simulink model "figura10"  (Simulink 8.8)
settings: Solver=ode45  StartTime=0.0  RelTol=1e-3  EnableMultiTasking=on
libraries: dsparch4 x1, dspsrcs4 x1
settings Model: Creator=chritian  LastModifiedBy=HP
settings OptimizationCC: ExpressionDepthLimit=2147483647  InitFltsAndDblsToZero=on
settings DebuggingCC: SolverPrmCheckMsg=warning  StrictBusMsg=Warning
settings GRTTargetCC: GeneratePreprocessorConditionals=Use local settings

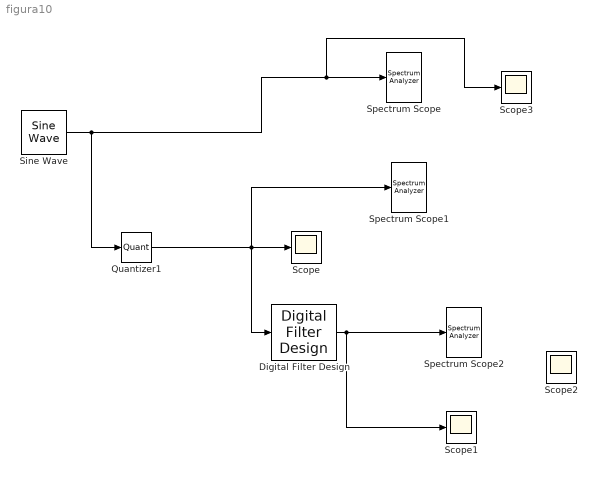
== system figura10 ==
  Digital Filter Design : dsparch4/Digital Filter Design  mwdsp_browser_bugfix_var=off
  Quantizer1 : Quantizer
  Scope{,1..3} (4 alike) : Scope
  Sine Wave : dspsrcs4/Sine Wave  Amplitude=1  Frequency=100  Phase=0  SampleMode=Discrete  OutComplex=Real  CompMethod=Trigonometric fcn  TableSize=Speed  SampleTime=1/1000  SamplesPerFrame=1  ResetState=Restart at time zero  OutputFrames=on  dataType=double  wordLen=16  udDataType=sfix(16)  fracBitsMode=Best precision  numFracBits=15  OutDataTypeStr=double  LastOutDataTypeStr=double
  Spectrum Scope : SpectrumAnalyzer
  Spectrum Scope1 : SpectrumAnalyzer
  Spectrum Scope2 : SpectrumAnalyzer
  wires:
  Sine Wave/1 -> Quantizer1/1, Scope3/1, Spectrum Scope/1
  Quantizer1/1 -> Scope/1, Spectrum Scope1/1, Digital Filter Design/1
  Digital Filter Design/1 -> Scope1/1, Spectrum Scope2/1
